simulink model "c00017M_harness"  (R2018a)
settings: Solver=FixedStepAuto  StartTime=0.0  StopTime=300  FixedStep=0.1  RelTol=1e-3
undefined symbols (not defined in the file): A1, hmax, R1, R2, sigbuilder_block
(part 2 of 6)

== system c00017M_harness/M127 ==
  note: VALUES
      | ---------------------------------
      | ControlType = 1 | 2 | 3
      | FillTank = 0 | 1
      | EmptyTank = 0 | 1
      | ManualReference between 0 and 1
      | Tempreature between 0 and 100
      | EmergencyButton = 0 | 1
      | LiquidLevel between 0 and 1 (hmax)
  note: Inputs For Tank2
  note: NAMES
      | --------------------------------------------
      | CT1 = ControlType Tank 1
      | F1 = Fill Tank 1
      | E1 = Empty Tank 1
      | MR1 = Manual Reference Tank1
      | T1 = Temperature Tank 1
      | EB1 = Emergency Button Tank 1
      | LL1 = Liquid Level 1
  note: Inputs For Tank3
  note: Inputs For Tank1
  CT2 : Inport
  F2 : Inport  Port=2
  E2 : Inport  Port=3
  MR2 : Inport  Port=4
  T2 : Inport  Port=5
  EB2 : Inport  Port=6
  Tank2 : Subsystem
  LL2 : Outport
  wires:
  Tank2/1(LL2) -> LL2/1
  EB2/1 -> Tank2/6(EB2)
  CT2/1 -> Tank2/1(CT2)
  F2/1 -> Tank2/2(F2)
  E2/1 -> Tank2/3(E2)
  T2/1 -> Tank2/5(T2)
  MR2/1 -> Tank2/4(MR2)

== system c00017M_harness/M128 ==
  note: VALUES
      | ---------------------------------
      | ControlType = 1 | 2 | 3
      | FillTank = 0 | 1
      | EmptyTank = 0 | 1
      | ManualReference between 0 and 1
      | Tempreature between 0 and 100
      | EmergencyButton = 0 | 1
      | LiquidLevel between 0 and 1 (hmax)
  note: Inputs For Tank2
  note: NAMES
      | --------------------------------------------
      | CT1 = ControlType Tank 1
      | F1 = Fill Tank 1
      | E1 = Empty Tank 1
      | MR1 = Manual Reference Tank1
      | T1 = Temperature Tank 1
      | EB1 = Emergency Button Tank 1
      | LL1 = Liquid Level 1
  note: Inputs For Tank3
  note: Inputs For Tank1
  CT2 : Inport
  F2 : Inport  Port=2
  E2 : Inport  Port=3
  MR2 : Inport  Port=4
  T2 : Inport  Port=5
  EB2 : Inport  Port=6
  Tank2 : Subsystem
  LL2 : Outport
  wires:
  Tank2/1(LL2) -> LL2/1
  EB2/1 -> Tank2/6(EB2)
  CT2/1 -> Tank2/1(CT2)
  F2/1 -> Tank2/2(F2)
  E2/1 -> Tank2/3(E2)
  T2/1 -> Tank2/5(T2)
  MR2/1 -> Tank2/4(MR2)

== system c00017M_harness/M129 ==
  note: VALUES
      | ---------------------------------
      | ControlType = 1 | 2 | 3
      | FillTank = 0 | 1
      | EmptyTank = 0 | 1
      | ManualReference between 0 and 1
      | Tempreature between 0 and 100
      | EmergencyButton = 0 | 1
      | LiquidLevel between 0 and 1 (hmax)
  note: Inputs For Tank2
  note: NAMES
      | --------------------------------------------
      | CT1 = ControlType Tank 1
      | F1 = Fill Tank 1
      | E1 = Empty Tank 1
      | MR1 = Manual Reference Tank1
      | T1 = Temperature Tank 1
      | EB1 = Emergency Button Tank 1
      | LL1 = Liquid Level 1
  note: Inputs For Tank3
  note: Inputs For Tank1
  CT2 : Inport
  F2 : Inport  Port=2
  E2 : Inport  Port=3
  MR2 : Inport  Port=4
  T2 : Inport  Port=5
  EB2 : Inport  Port=6
  Tank2 : Subsystem
  LL2 : Outport
  wires:
  Tank2/1(LL2) -> LL2/1
  EB2/1 -> Tank2/6(EB2)
  CT2/1 -> Tank2/1(CT2)
  F2/1 -> Tank2/2(F2)
  E2/1 -> Tank2/3(E2)
  T2/1 -> Tank2/5(T2)
  MR2/1 -> Tank2/4(MR2)

== system c00017M_harness/M130 ==
  note: VALUES
      | ---------------------------------
      | ControlType = 1 | 2 | 3
      | FillTank = 0 | 1
      | EmptyTank = 0 | 1
      | ManualReference between 0 and 1
      | Tempreature between 0 and 100
      | EmergencyButton = 0 | 1
      | LiquidLevel between 0 and 1 (hmax)
  note: Inputs For Tank2
  note: NAMES
      | --------------------------------------------
      | CT1 = ControlType Tank 1
      | F1 = Fill Tank 1
      | E1 = Empty Tank 1
      | MR1 = Manual Reference Tank1
      | T1 = Temperature Tank 1
      | EB1 = Emergency Button Tank 1
      | LL1 = Liquid Level 1
  note: Inputs For Tank3
  note: Inputs For Tank1
  CT2 : Inport
  F2 : Inport  Port=2
  E2 : Inport  Port=3
  MR2 : Inport  Port=4
  T2 : Inport  Port=5
  EB2 : Inport  Port=6
  Tank2 : Subsystem
  LL2 : Outport
  wires:
  Tank2/1(LL2) -> LL2/1
  EB2/1 -> Tank2/6(EB2)
  CT2/1 -> Tank2/1(CT2)
  F2/1 -> Tank2/2(F2)
  E2/1 -> Tank2/3(E2)
  T2/1 -> Tank2/5(T2)
  MR2/1 -> Tank2/4(MR2)

== system c00017M_harness/M131 ==
  note: VALUES
      | ---------------------------------
      | ControlType = 1 | 2 | 3
      | FillTank = 0 | 1
      | EmptyTank = 0 | 1
      | ManualReference between 0 and 1
      | Tempreature between 0 and 100
      | EmergencyButton = 0 | 1
      | LiquidLevel between 0 and 1 (hmax)
  note: Inputs For Tank2
  note: NAMES
      | --------------------------------------------
      | CT1 = ControlType Tank 1
      | F1 = Fill Tank 1
      | E1 = Empty Tank 1
      | MR1 = Manual Reference Tank1
      | T1 = Temperature Tank 1
      | EB1 = Emergency Button Tank 1
      | LL1 = Liquid Level 1
  note: Inputs For Tank3
  note: Inputs For Tank1
  CT2 : Inport
  F2 : Inport  Port=2
  E2 : Inport  Port=3
  MR2 : Inport  Port=4
  T2 : Inport  Port=5
  EB2 : Inport  Port=6
  Tank2 : Subsystem
  LL2 : Outport
  wires:
  Tank2/1(LL2) -> LL2/1
  EB2/1 -> Tank2/6(EB2)
  CT2/1 -> Tank2/1(CT2)
  F2/1 -> Tank2/2(F2)
  E2/1 -> Tank2/3(E2)
  T2/1 -> Tank2/5(T2)
  MR2/1 -> Tank2/4(MR2)

== system c00017M_harness/M132 ==
  note: VALUES
      | ---------------------------------
      | ControlType = 1 | 2 | 3
      | FillTank = 0 | 1
      | EmptyTank = 0 | 1
      | ManualReference between 0 and 1
      | Tempreature between 0 and 100
      | EmergencyButton = 0 | 1
      | LiquidLevel between 0 and 1 (hmax)
  note: Inputs For Tank2
  note: NAMES
      | --------------------------------------------
      | CT1 = ControlType Tank 1
      | F1 = Fill Tank 1
      | E1 = Empty Tank 1
      | MR1 = Manual Reference Tank1
      | T1 = Temperature Tank 1
      | EB1 = Emergency Button Tank 1
      | LL1 = Liquid Level 1
  note: Inputs For Tank3
  note: Inputs For Tank1
  CT2 : Inport
  F2 : Inport  Port=2
  E2 : Inport  Port=3
  MR2 : Inport  Port=4
  T2 : Inport  Port=5
  EB2 : Inport  Port=6
  Tank2 : Subsystem
  LL2 : Outport
  wires:
  Tank2/1(LL2) -> LL2/1
  EB2/1 -> Tank2/6(EB2)
  CT2/1 -> Tank2/1(CT2)
  F2/1 -> Tank2/2(F2)
  E2/1 -> Tank2/3(E2)
  T2/1 -> Tank2/5(T2)
  MR2/1 -> Tank2/4(MR2)

== system c00017M_harness/M133 ==
  note: VALUES
      | ---------------------------------
      | ControlType = 1 | 2 | 3
      | FillTank = 0 | 1
      | EmptyTank = 0 | 1
      | ManualReference between 0 and 1
      | Tempreature between 0 and 100
      | EmergencyButton = 0 | 1
      | LiquidLevel between 0 and 1 (hmax)
  note: Inputs For Tank2
  note: NAMES
      | --------------------------------------------
      | CT1 = ControlType Tank 1
      | F1 = Fill Tank 1
      | E1 = Empty Tank 1
      | MR1 = Manual Reference Tank1
      | T1 = Temperature Tank 1
      | EB1 = Emergency Button Tank 1
      | LL1 = Liquid Level 1
  note: Inputs For Tank3
  note: Inputs For Tank1
  CT2 : Inport
  F2 : Inport  Port=2
  E2 : Inport  Port=3
  MR2 : Inport  Port=4
  T2 : Inport  Port=5
  EB2 : Inport  Port=6
  Tank2 : Subsystem
  LL2 : Outport
  wires:
  Tank2/1(LL2) -> LL2/1
  EB2/1 -> Tank2/6(EB2)
  CT2/1 -> Tank2/1(CT2)
  F2/1 -> Tank2/2(F2)
  E2/1 -> Tank2/3(E2)
  T2/1 -> Tank2/5(T2)
  MR2/1 -> Tank2/4(MR2)

== system c00017M_harness/M134 ==
  note: VALUES
      | ---------------------------------
      | ControlType = 1 | 2 | 3
      | FillTank = 0 | 1
      | EmptyTank = 0 | 1
      | ManualReference between 0 and 1
      | Tempreature between 0 and 100
      | EmergencyButton = 0 | 1
      | LiquidLevel between 0 and 1 (hmax)
  note: Inputs For Tank2
  note: NAMES
      | --------------------------------------------
      | CT1 = ControlType Tank 1
      | F1 = Fill Tank 1
      | E1 = Empty Tank 1
      | MR1 = Manual Reference Tank1
      | T1 = Temperature Tank 1
      | EB1 = Emergency Button Tank 1
      | LL1 = Liquid Level 1
  note: Inputs For Tank3
  note: Inputs For Tank1
  CT2 : Inport
  F2 : Inport  Port=2
  E2 : Inport  Port=3
  MR2 : Inport  Port=4
  T2 : Inport  Port=5
  EB2 : Inport  Port=6
  Tank2 : Subsystem
  LL2 : Outport
  wires:
  Tank2/1(LL2) -> LL2/1
  EB2/1 -> Tank2/6(EB2)
  CT2/1 -> Tank2/1(CT2)
  F2/1 -> Tank2/2(F2)
  E2/1 -> Tank2/3(E2)
  T2/1 -> Tank2/5(T2)
  MR2/1 -> Tank2/4(MR2)

== system c00017M_harness/M135 ==
  note: VALUES
      | ---------------------------------
      | ControlType = 1 | 2 | 3
      | FillTank = 0 | 1
      | EmptyTank = 0 | 1
      | ManualReference between 0 and 1
      | Tempreature between 0 and 100
      | EmergencyButton = 0 | 1
      | LiquidLevel between 0 and 1 (hmax)
  note: Inputs For Tank2
  note: NAMES
      | --------------------------------------------
      | CT1 = ControlType Tank 1
      | F1 = Fill Tank 1
      | E1 = Empty Tank 1
      | MR1 = Manual Reference Tank1
      | T1 = Temperature Tank 1
      | EB1 = Emergency Button Tank 1
      | LL1 = Liquid Level 1
  note: Inputs For Tank3
  note: Inputs For Tank1
  CT2 : Inport
  F2 : Inport  Port=2
  E2 : Inport  Port=3
  MR2 : Inport  Port=4
  T2 : Inport  Port=5
  EB2 : Inport  Port=6
  Tank2 : Subsystem
  LL2 : Outport
  wires:
  Tank2/1(LL2) -> LL2/1
  EB2/1 -> Tank2/6(EB2)
  CT2/1 -> Tank2/1(CT2)
  F2/1 -> Tank2/2(F2)
  E2/1 -> Tank2/3(E2)
  T2/1 -> Tank2/5(T2)
  MR2/1 -> Tank2/4(MR2)

== system c00017M_harness/M136 ==
  note: VALUES
      | ---------------------------------
      | ControlType = 1 | 2 | 3
      | FillTank = 0 | 1
      | EmptyTank = 0 | 1
      | ManualReference between 0 and 1
      | Tempreature between 0 and 100
      | EmergencyButton = 0 | 1
      | LiquidLevel between 0 and 1 (hmax)
  note: Inputs For Tank2
  note: NAMES
      | --------------------------------------------
      | CT1 = ControlType Tank 1
      | F1 = Fill Tank 1
      | E1 = Empty Tank 1
      | MR1 = Manual Reference Tank1
      | T1 = Temperature Tank 1
      | EB1 = Emergency Button Tank 1
      | LL1 = Liquid Level 1
  note: Inputs For Tank3
  note: Inputs For Tank1
  CT2 : Inport
  F2 : Inport  Port=2
  E2 : Inport  Port=3
  MR2 : Inport  Port=4
  T2 : Inport  Port=5
  EB2 : Inport  Port=6
  Tank2 : Subsystem
  LL2 : Outport
  wires:
  Tank2/1(LL2) -> LL2/1
  EB2/1 -> Tank2/6(EB2)
  CT2/1 -> Tank2/1(CT2)
  F2/1 -> Tank2/2(F2)
  E2/1 -> Tank2/3(E2)
  T2/1 -> Tank2/5(T2)
  MR2/1 -> Tank2/4(MR2)

== system c00017M_harness/M137 ==
  note: VALUES
      | ---------------------------------
      | ControlType = 1 | 2 | 3
      | FillTank = 0 | 1
      | EmptyTank = 0 | 1
      | ManualReference between 0 and 1
      | Tempreature between 0 and 100
      | EmergencyButton = 0 | 1
      | LiquidLevel between 0 and 1 (hmax)
  note: Inputs For Tank2
  note: NAMES
      | --------------------------------------------
      | CT1 = ControlType Tank 1
      | F1 = Fill Tank 1
      | E1 = Empty Tank 1
      | MR1 = Manual Reference Tank1
      | T1 = Temperature Tank 1
      | EB1 = Emergency Button Tank 1
      | LL1 = Liquid Level 1
  note: Inputs For Tank3
  note: Inputs For Tank1
  CT2 : Inport
  F2 : Inport  Port=2
  E2 : Inport  Port=3
  MR2 : Inport  Port=4
  T2 : Inport  Port=5
  EB2 : Inport  Port=6
  Tank2 : Subsystem
  LL2 : Outport
  wires:
  Tank2/1(LL2) -> LL2/1
  EB2/1 -> Tank2/6(EB2)
  CT2/1 -> Tank2/1(CT2)
  F2/1 -> Tank2/2(F2)
  E2/1 -> Tank2/3(E2)
  T2/1 -> Tank2/5(T2)
  MR2/1 -> Tank2/4(MR2)

== system c00017M_harness/M138 ==
  note: VALUES
      | ---------------------------------
      | ControlType = 1 | 2 | 3
      | FillTank = 0 | 1
      | EmptyTank = 0 | 1
      | ManualReference between 0 and 1
      | Tempreature between 0 and 100
      | EmergencyButton = 0 | 1
      | LiquidLevel between 0 and 1 (hmax)
  note: Inputs For Tank2
  note: NAMES
      | --------------------------------------------
      | CT1 = ControlType Tank 1
      | F1 = Fill Tank 1
      | E1 = Empty Tank 1
      | MR1 = Manual Reference Tank1
      | T1 = Temperature Tank 1
      | EB1 = Emergency Button Tank 1
      | LL1 = Liquid Level 1
  note: Inputs For Tank3
  note: Inputs For Tank1
  CT2 : Inport
  F2 : Inport  Port=2
  E2 : Inport  Port=3
  MR2 : Inport  Port=4
  T2 : Inport  Port=5
  EB2 : Inport  Port=6
  Tank2 : Subsystem
  LL2 : Outport
  wires:
  Tank2/1(LL2) -> LL2/1
  EB2/1 -> Tank2/6(EB2)
  CT2/1 -> Tank2/1(CT2)
  F2/1 -> Tank2/2(F2)
  E2/1 -> Tank2/3(E2)
  T2/1 -> Tank2/5(T2)
  MR2/1 -> Tank2/4(MR2)

== system c00017M_harness/M140 ==
  note: VALUES
      | ---------------------------------
      | ControlType = 1 | 2 | 3
      | FillTank = 0 | 1
      | EmptyTank = 0 | 1
      | ManualReference between 0 and 1
      | Tempreature between 0 and 100
      | EmergencyButton = 0 | 1
      | LiquidLevel between 0 and 1 (hmax)
  note: Inputs For Tank2
  note: NAMES
      | --------------------------------------------
      | CT1 = ControlType Tank 1
      | F1 = Fill Tank 1
      | E1 = Empty Tank 1
      | MR1 = Manual Reference Tank1
      | T1 = Temperature Tank 1
      | EB1 = Emergency Button Tank 1
      | LL1 = Liquid Level 1
  note: Inputs For Tank3
  note: Inputs For Tank1
  CT2 : Inport
  F2 : Inport  Port=2
  E2 : Inport  Port=3
  MR2 : Inport  Port=4
  T2 : Inport  Port=5
  EB2 : Inport  Port=6
  Tank2 : Subsystem
  LL2 : Outport
  wires:
  Tank2/1(LL2) -> LL2/1
  EB2/1 -> Tank2/6(EB2)
  CT2/1 -> Tank2/1(CT2)
  F2/1 -> Tank2/2(F2)
  E2/1 -> Tank2/3(E2)
  T2/1 -> Tank2/5(T2)
  MR2/1 -> Tank2/4(MR2)

== system c00017M_harness/M141 ==
  note: VALUES
      | ---------------------------------
      | ControlType = 1 | 2 | 3
      | FillTank = 0 | 1
      | EmptyTank = 0 | 1
      | ManualReference between 0 and 1
      | Tempreature between 0 and 100
      | EmergencyButton = 0 | 1
      | LiquidLevel between 0 and 1 (hmax)
  note: Inputs For Tank2
  note: NAMES
      | --------------------------------------------
      | CT1 = ControlType Tank 1
      | F1 = Fill Tank 1
      | E1 = Empty Tank 1
      | MR1 = Manual Reference Tank1
      | T1 = Temperature Tank 1
      | EB1 = Emergency Button Tank 1
      | LL1 = Liquid Level 1
  note: Inputs For Tank3
  note: Inputs For Tank1
  CT2 : Inport
  F2 : Inport  Port=2
  E2 : Inport  Port=3
  MR2 : Inport  Port=4
  T2 : Inport  Port=5
  EB2 : Inport  Port=6
  Tank2 : Subsystem
  LL2 : Outport
  wires:
  Tank2/1(LL2) -> LL2/1
  EB2/1 -> Tank2/6(EB2)
  CT2/1 -> Tank2/1(CT2)
  F2/1 -> Tank2/2(F2)
  E2/1 -> Tank2/3(E2)
  T2/1 -> Tank2/5(T2)
  MR2/1 -> Tank2/4(MR2)

== system c00017M_harness/M142 ==
  note: VALUES
      | ---------------------------------
      | ControlType = 1 | 2 | 3
      | FillTank = 0 | 1
      | EmptyTank = 0 | 1
      | ManualReference between 0 and 1
      | Tempreature between 0 and 100
      | EmergencyButton = 0 | 1
      | LiquidLevel between 0 and 1 (hmax)
  note: Inputs For Tank2
  note: NAMES
      | --------------------------------------------
      | CT1 = ControlType Tank 1
      | F1 = Fill Tank 1
      | E1 = Empty Tank 1
      | MR1 = Manual Reference Tank1
      | T1 = Temperature Tank 1
      | EB1 = Emergency Button Tank 1
      | LL1 = Liquid Level 1
  note: Inputs For Tank3
  note: Inputs For Tank1
  CT2 : Inport
  F2 : Inport  Port=2
  E2 : Inport  Port=3
  MR2 : Inport  Port=4
  T2 : Inport  Port=5
  EB2 : Inport  Port=6
  Tank2 : Subsystem
  LL2 : Outport
  wires:
  Tank2/1(LL2) -> LL2/1
  EB2/1 -> Tank2/6(EB2)
  CT2/1 -> Tank2/1(CT2)
  F2/1 -> Tank2/2(F2)
  E2/1 -> Tank2/3(E2)
  T2/1 -> Tank2/5(T2)
  MR2/1 -> Tank2/4(MR2)

== system c00017M_harness/M143 ==
  note: VALUES
      | ---------------------------------
      | ControlType = 1 | 2 | 3
      | FillTank = 0 | 1
      | EmptyTank = 0 | 1
      | ManualReference between 0 and 1
      | Tempreature between 0 and 100
      | EmergencyButton = 0 | 1
      | LiquidLevel between 0 and 1 (hmax)
  note: Inputs For Tank2
  note: NAMES
      | --------------------------------------------
      | CT1 = ControlType Tank 1
      | F1 = Fill Tank 1
      | E1 = Empty Tank 1
      | MR1 = Manual Reference Tank1
      | T1 = Temperature Tank 1
      | EB1 = Emergency Button Tank 1
      | LL1 = Liquid Level 1
  note: Inputs For Tank3
  note: Inputs For Tank1
  CT2 : Inport
  F2 : Inport  Port=2
  E2 : Inport  Port=3
  MR2 : Inport  Port=4
  T2 : Inport  Port=5
  EB2 : Inport  Port=6
  Tank2 : Subsystem
  LL2 : Outport
  wires:
  Tank2/1(LL2) -> LL2/1
  EB2/1 -> Tank2/6(EB2)
  CT2/1 -> Tank2/1(CT2)
  F2/1 -> Tank2/2(F2)
  E2/1 -> Tank2/3(E2)
  T2/1 -> Tank2/5(T2)
  MR2/1 -> Tank2/4(MR2)

== system c00017M_harness/M151 ==
  note: VALUES
      | ---------------------------------
      | ControlType = 1 | 2 | 3
      | FillTank = 0 | 1
      | EmptyTank = 0 | 1
      | ManualReference between 0 and 1
      | Tempreature between 0 and 100
      | EmergencyButton = 0 | 1
      | LiquidLevel between 0 and 1 (hmax)
  note: Inputs For Tank2
  note: NAMES
      | --------------------------------------------
      | CT1 = ControlType Tank 1
      | F1 = Fill Tank 1
      | E1 = Empty Tank 1
      | MR1 = Manual Reference Tank1
      | T1 = Temperature Tank 1
      | EB1 = Emergency Button Tank 1
      | LL1 = Liquid Level 1
  note: Inputs For Tank3
  note: Inputs For Tank1
  CT2 : Inport
  F2 : Inport  Port=2
  E2 : Inport  Port=3
  MR2 : Inport  Port=4
  T2 : Inport  Port=5
  EB2 : Inport  Port=6
  Tank2 : Subsystem
  LL2 : Outport
  wires:
  Tank2/1(LL2) -> LL2/1
  EB2/1 -> Tank2/6(EB2)
  CT2/1 -> Tank2/1(CT2)
  F2/1 -> Tank2/2(F2)
  E2/1 -> Tank2/3(E2)
  T2/1 -> Tank2/5(T2)
  MR2/1 -> Tank2/4(MR2)

== system c00017M_harness/M152 ==
  note: VALUES
      | ---------------------------------
      | ControlType = 1 | 2 | 3
      | FillTank = 0 | 1
      | EmptyTank = 0 | 1
      | ManualReference between 0 and 1
      | Tempreature between 0 and 100
      | EmergencyButton = 0 | 1
      | LiquidLevel between 0 and 1 (hmax)
  note: Inputs For Tank2
  note: NAMES
      | --------------------------------------------
      | CT1 = ControlType Tank 1
      | F1 = Fill Tank 1
      | E1 = Empty Tank 1
      | MR1 = Manual Reference Tank1
      | T1 = Temperature Tank 1
      | EB1 = Emergency Button Tank 1
      | LL1 = Liquid Level 1
  note: Inputs For Tank3
  note: Inputs For Tank1
  CT2 : Inport
  F2 : Inport  Port=2
  E2 : Inport  Port=3
  MR2 : Inport  Port=4
  T2 : Inport  Port=5
  EB2 : Inport  Port=6
  Tank2 : Subsystem
  LL2 : Outport
  wires:
  Tank2/1(LL2) -> LL2/1
  EB2/1 -> Tank2/6(EB2)
  CT2/1 -> Tank2/1(CT2)
  F2/1 -> Tank2/2(F2)
  E2/1 -> Tank2/3(E2)
  T2/1 -> Tank2/5(T2)
  MR2/1 -> Tank2/4(MR2)

== system c00017M_harness/M153 ==
  note: VALUES
      | ---------------------------------
      | ControlType = 1 | 2 | 3
      | FillTank = 0 | 1
      | EmptyTank = 0 | 1
      | ManualReference between 0 and 1
      | Tempreature between 0 and 100
      | EmergencyButton = 0 | 1
      | LiquidLevel between 0 and 1 (hmax)
  note: Inputs For Tank2
  note: NAMES
      | --------------------------------------------
      | CT1 = ControlType Tank 1
      | F1 = Fill Tank 1
      | E1 = Empty Tank 1
      | MR1 = Manual Reference Tank1
      | T1 = Temperature Tank 1
      | EB1 = Emergency Button Tank 1
      | LL1 = Liquid Level 1
  note: Inputs For Tank3
  note: Inputs For Tank1
  CT2 : Inport
  F2 : Inport  Port=2
  E2 : Inport  Port=3
  MR2 : Inport  Port=4
  T2 : Inport  Port=5
  EB2 : Inport  Port=6
  Tank2 : Subsystem
  LL2 : Outport
  wires:
  Tank2/1(LL2) -> LL2/1
  EB2/1 -> Tank2/6(EB2)
  CT2/1 -> Tank2/1(CT2)
  F2/1 -> Tank2/2(F2)
  E2/1 -> Tank2/3(E2)
  T2/1 -> Tank2/5(T2)
  MR2/1 -> Tank2/4(MR2)

== system c00017M_harness/M154 ==
  note: VALUES
      | ---------------------------------
      | ControlType = 1 | 2 | 3
      | FillTank = 0 | 1
      | EmptyTank = 0 | 1
      | ManualReference between 0 and 1
      | Tempreature between 0 and 100
      | EmergencyButton = 0 | 1
      | LiquidLevel between 0 and 1 (hmax)
  note: Inputs For Tank2
  note: NAMES
      | --------------------------------------------
      | CT1 = ControlType Tank 1
      | F1 = Fill Tank 1
      | E1 = Empty Tank 1
      | MR1 = Manual Reference Tank1
      | T1 = Temperature Tank 1
      | EB1 = Emergency Button Tank 1
      | LL1 = Liquid Level 1
  note: Inputs For Tank3
  note: Inputs For Tank1
  CT2 : Inport
  F2 : Inport  Port=2
  E2 : Inport  Port=3
  MR2 : Inport  Port=4
  T2 : Inport  Port=5
  EB2 : Inport  Port=6
  Tank2 : Subsystem
  LL2 : Outport
  wires:
  Tank2/1(LL2) -> LL2/1
  EB2/1 -> Tank2/6(EB2)
  CT2/1 -> Tank2/1(CT2)
  F2/1 -> Tank2/2(F2)
  E2/1 -> Tank2/3(E2)
  T2/1 -> Tank2/5(T2)
  MR2/1 -> Tank2/4(MR2)

== system c00017M_harness/M155 ==
  note: VALUES
      | ---------------------------------
      | ControlType = 1 | 2 | 3
      | FillTank = 0 | 1
      | EmptyTank = 0 | 1
      | ManualReference between 0 and 1
      | Tempreature between 0 and 100
      | EmergencyButton = 0 | 1
      | LiquidLevel between 0 and 1 (hmax)
  note: Inputs For Tank2
  note: NAMES
      | --------------------------------------------
      | CT1 = ControlType Tank 1
      | F1 = Fill Tank 1
      | E1 = Empty Tank 1
      | MR1 = Manual Reference Tank1
      | T1 = Temperature Tank 1
      | EB1 = Emergency Button Tank 1
      | LL1 = Liquid Level 1
  note: Inputs For Tank3
  note: Inputs For Tank1
  CT2 : Inport
  F2 : Inport  Port=2
  E2 : Inport  Port=3
  MR2 : Inport  Port=4
  T2 : Inport  Port=5
  EB2 : Inport  Port=6
  Tank2 : Subsystem
  LL2 : Outport
  wires:
  Tank2/1(LL2) -> LL2/1
  EB2/1 -> Tank2/6(EB2)
  CT2/1 -> Tank2/1(CT2)
  F2/1 -> Tank2/2(F2)
  E2/1 -> Tank2/3(E2)
  T2/1 -> Tank2/5(T2)
  MR2/1 -> Tank2/4(MR2)

== system c00017M_harness/M156 ==
  note: VALUES
      | ---------------------------------
      | ControlType = 1 | 2 | 3
      | FillTank = 0 | 1
      | EmptyTank = 0 | 1
      | ManualReference between 0 and 1
      | Tempreature between 0 and 100
      | EmergencyButton = 0 | 1
      | LiquidLevel between 0 and 1 (hmax)
  note: Inputs For Tank2
  note: NAMES
      | --------------------------------------------
      | CT1 = ControlType Tank 1
      | F1 = Fill Tank 1
      | E1 = Empty Tank 1
      | MR1 = Manual Reference Tank1
      | T1 = Temperature Tank 1
      | EB1 = Emergency Button Tank 1
      | LL1 = Liquid Level 1
  note: Inputs For Tank3
  note: Inputs For Tank1
  CT2 : Inport
  F2 : Inport  Port=2
  E2 : Inport  Port=3
  MR2 : Inport  Port=4
  T2 : Inport  Port=5
  EB2 : Inport  Port=6
  Tank2 : Subsystem
  LL2 : Outport
  wires:
  Tank2/1(LL2) -> LL2/1
  EB2/1 -> Tank2/6(EB2)
  CT2/1 -> Tank2/1(CT2)
  F2/1 -> Tank2/2(F2)
  E2/1 -> Tank2/3(E2)
  T2/1 -> Tank2/5(T2)
  MR2/1 -> Tank2/4(MR2)

== system c00017M_harness/M157 ==
  note: VALUES
      | ---------------------------------
      | ControlType = 1 | 2 | 3
      | FillTank = 0 | 1
      | EmptyTank = 0 | 1
      | ManualReference between 0 and 1
      | Tempreature between 0 and 100
      | EmergencyButton = 0 | 1
      | LiquidLevel between 0 and 1 (hmax)
  note: Inputs For Tank2
  note: NAMES
      | --------------------------------------------
      | CT1 = ControlType Tank 1
      | F1 = Fill Tank 1
      | E1 = Empty Tank 1
      | MR1 = Manual Reference Tank1
      | T1 = Temperature Tank 1
      | EB1 = Emergency Button Tank 1
      | LL1 = Liquid Level 1
  note: Inputs For Tank3
  note: Inputs For Tank1
  CT2 : Inport
  F2 : Inport  Port=2
  E2 : Inport  Port=3
  MR2 : Inport  Port=4
  T2 : Inport  Port=5
  EB2 : Inport  Port=6
  Tank2 : Subsystem
  LL2 : Outport
  wires:
  Tank2/1(LL2) -> LL2/1
  EB2/1 -> Tank2/6(EB2)
  CT2/1 -> Tank2/1(CT2)
  F2/1 -> Tank2/2(F2)
  E2/1 -> Tank2/3(E2)
  T2/1 -> Tank2/5(T2)
  MR2/1 -> Tank2/4(MR2)

== system c00017M_harness/M158 ==
  note: VALUES
      | ---------------------------------
      | ControlType = 1 | 2 | 3
      | FillTank = 0 | 1
      | EmptyTank = 0 | 1
      | ManualReference between 0 and 1
      | Tempreature between 0 and 100
      | EmergencyButton = 0 | 1
      | LiquidLevel between 0 and 1 (hmax)
  note: Inputs For Tank2
  note: NAMES
      | --------------------------------------------
      | CT1 = ControlType Tank 1
      | F1 = Fill Tank 1
      | E1 = Empty Tank 1
      | MR1 = Manual Reference Tank1
      | T1 = Temperature Tank 1
      | EB1 = Emergency Button Tank 1
      | LL1 = Liquid Level 1
  note: Inputs For Tank3
  note: Inputs For Tank1
  CT2 : Inport
  F2 : Inport  Port=2
  E2 : Inport  Port=3
  MR2 : Inport  Port=4
  T2 : Inport  Port=5
  EB2 : Inport  Port=6
  Tank2 : Subsystem
  LL2 : Outport
  wires:
  Tank2/1(LL2) -> LL2/1
  EB2/1 -> Tank2/6(EB2)
  CT2/1 -> Tank2/1(CT2)
  F2/1 -> Tank2/2(F2)
  E2/1 -> Tank2/3(E2)
  T2/1 -> Tank2/5(T2)
  MR2/1 -> Tank2/4(MR2)

== system c00017M_harness/M159 ==
  note: VALUES
      | ---------------------------------
      | ControlType = 1 | 2 | 3
      | FillTank = 0 | 1
      | EmptyTank = 0 | 1
      | ManualReference between 0 and 1
      | Tempreature between 0 and 100
      | EmergencyButton = 0 | 1
      | LiquidLevel between 0 and 1 (hmax)
  note: Inputs For Tank2
  note: NAMES
      | --------------------------------------------
      | CT1 = ControlType Tank 1
      | F1 = Fill Tank 1
      | E1 = Empty Tank 1
      | MR1 = Manual Reference Tank1
      | T1 = Temperature Tank 1
      | EB1 = Emergency Button Tank 1
      | LL1 = Liquid Level 1
  note: Inputs For Tank3
  note: Inputs For Tank1
  CT2 : Inport
  F2 : Inport  Port=2
  E2 : Inport  Port=3
  MR2 : Inport  Port=4
  T2 : Inport  Port=5
  EB2 : Inport  Port=6
  Tank2 : Subsystem
  LL2 : Outport
  wires:
  Tank2/1(LL2) -> LL2/1
  EB2/1 -> Tank2/6(EB2)
  CT2/1 -> Tank2/1(CT2)
  F2/1 -> Tank2/2(F2)
  E2/1 -> Tank2/3(E2)
  T2/1 -> Tank2/5(T2)
  MR2/1 -> Tank2/4(MR2)

== system c00017M_harness/M160 ==
  note: VALUES
      | ---------------------------------
      | ControlType = 1 | 2 | 3
      | FillTank = 0 | 1
      | EmptyTank = 0 | 1
      | ManualReference between 0 and 1
      | Tempreature between 0 and 100
      | EmergencyButton = 0 | 1
      | LiquidLevel between 0 and 1 (hmax)
  note: Inputs For Tank2
  note: NAMES
      | --------------------------------------------
      | CT1 = ControlType Tank 1
      | F1 = Fill Tank 1
      | E1 = Empty Tank 1
      | MR1 = Manual Reference Tank1
      | T1 = Temperature Tank 1
      | EB1 = Emergency Button Tank 1
      | LL1 = Liquid Level 1
  note: Inputs For Tank3
  note: Inputs For Tank1
  CT2 : Inport
  F2 : Inport  Port=2
  E2 : Inport  Port=3
  MR2 : Inport  Port=4
  T2 : Inport  Port=5
  EB2 : Inport  Port=6
  Tank2 : Subsystem
  LL2 : Outport
  wires:
  Tank2/1(LL2) -> LL2/1
  EB2/1 -> Tank2/6(EB2)
  CT2/1 -> Tank2/1(CT2)
  F2/1 -> Tank2/2(F2)
  E2/1 -> Tank2/3(E2)
  T2/1 -> Tank2/5(T2)
  MR2/1 -> Tank2/4(MR2)

== system c00017M_harness/M161 ==
  note: VALUES
      | ---------------------------------
      | ControlType = 1 | 2 | 3
      | FillTank = 0 | 1
      | EmptyTank = 0 | 1
      | ManualReference between 0 and 1
      | Tempreature between 0 and 100
      | EmergencyButton = 0 | 1
      | LiquidLevel between 0 and 1 (hmax)
  note: Inputs For Tank2
  note: NAMES
      | --------------------------------------------
      | CT1 = ControlType Tank 1
      | F1 = Fill Tank 1
      | E1 = Empty Tank 1
      | MR1 = Manual Reference Tank1
      | T1 = Temperature Tank 1
      | EB1 = Emergency Button Tank 1
      | LL1 = Liquid Level 1
  note: Inputs For Tank3
  note: Inputs For Tank1
  CT2 : Inport
  F2 : Inport  Port=2
  E2 : Inport  Port=3
  MR2 : Inport  Port=4
  T2 : Inport  Port=5
  EB2 : Inport  Port=6
  Tank2 : Subsystem
  LL2 : Outport
  wires:
  Tank2/1(LL2) -> LL2/1
  EB2/1 -> Tank2/6(EB2)
  CT2/1 -> Tank2/1(CT2)
  F2/1 -> Tank2/2(F2)
  E2/1 -> Tank2/3(E2)
  T2/1 -> Tank2/5(T2)
  MR2/1 -> Tank2/4(MR2)

== system c00017M_harness/M162 ==
  note: VALUES
      | ---------------------------------
      | ControlType = 1 | 2 | 3
      | FillTank = 0 | 1
      | EmptyTank = 0 | 1
      | ManualReference between 0 and 1
      | Tempreature between 0 and 100
      | EmergencyButton = 0 | 1
      | LiquidLevel between 0 and 1 (hmax)
  note: Inputs For Tank2
  note: NAMES
      | --------------------------------------------
      | CT1 = ControlType Tank 1
      | F1 = Fill Tank 1
      | E1 = Empty Tank 1
      | MR1 = Manual Reference Tank1
      | T1 = Temperature Tank 1
      | EB1 = Emergency Button Tank 1
      | LL1 = Liquid Level 1
  note: Inputs For Tank3
  note: Inputs For Tank1
  CT2 : Inport
  F2 : Inport  Port=2
  E2 : Inport  Port=3
  MR2 : Inport  Port=4
  T2 : Inport  Port=5
  EB2 : Inport  Port=6
  Tank2 : Subsystem
  LL2 : Outport
  wires:
  Tank2/1(LL2) -> LL2/1
  EB2/1 -> Tank2/6(EB2)
  CT2/1 -> Tank2/1(CT2)
  F2/1 -> Tank2/2(F2)
  E2/1 -> Tank2/3(E2)
  T2/1 -> Tank2/5(T2)
  MR2/1 -> Tank2/4(MR2)

== system c00017M_harness/M163 ==
  note: VALUES
      | ---------------------------------
      | ControlType = 1 | 2 | 3
      | FillTank = 0 | 1
      | EmptyTank = 0 | 1
      | ManualReference between 0 and 1
      | Tempreature between 0 and 100
      | EmergencyButton = 0 | 1
      | LiquidLevel between 0 and 1 (hmax)
  note: Inputs For Tank2
  note: NAMES
      | --------------------------------------------
      | CT1 = ControlType Tank 1
      | F1 = Fill Tank 1
      | E1 = Empty Tank 1
      | MR1 = Manual Reference Tank1
      | T1 = Temperature Tank 1
      | EB1 = Emergency Button Tank 1
      | LL1 = Liquid Level 1
  note: Inputs For Tank3
  note: Inputs For Tank1
  CT2 : Inport
  F2 : Inport  Port=2
  E2 : Inport  Port=3
  MR2 : Inport  Port=4
  T2 : Inport  Port=5
  EB2 : Inport  Port=6
  Tank2 : Subsystem
  LL2 : Outport
  wires:
  Tank2/1(LL2) -> LL2/1
  EB2/1 -> Tank2/6(EB2)
  CT2/1 -> Tank2/1(CT2)
  F2/1 -> Tank2/2(F2)
  E2/1 -> Tank2/3(E2)
  T2/1 -> Tank2/5(T2)
  MR2/1 -> Tank2/4(MR2)

== system c00017M_harness/M164 ==
  note: VALUES
      | ---------------------------------
      | ControlType = 1 | 2 | 3
      | FillTank = 0 | 1
      | EmptyTank = 0 | 1
      | ManualReference between 0 and 1
      | Tempreature between 0 and 100
      | EmergencyButton = 0 | 1
      | LiquidLevel between 0 and 1 (hmax)
  note: Inputs For Tank2
  note: NAMES
      | --------------------------------------------
      | CT1 = ControlType Tank 1
      | F1 = Fill Tank 1
      | E1 = Empty Tank 1
      | MR1 = Manual Reference Tank1
      | T1 = Temperature Tank 1
      | EB1 = Emergency Button Tank 1
      | LL1 = Liquid Level 1
  note: Inputs For Tank3
  note: Inputs For Tank1
  CT2 : Inport
  F2 : Inport  Port=2
  E2 : Inport  Port=3
  MR2 : Inport  Port=4
  T2 : Inport  Port=5
  EB2 : Inport  Port=6
  Tank2 : Subsystem
  LL2 : Outport
  wires:
  Tank2/1(LL2) -> LL2/1
  EB2/1 -> Tank2/6(EB2)
  CT2/1 -> Tank2/1(CT2)
  F2/1 -> Tank2/2(F2)
  E2/1 -> Tank2/3(E2)
  T2/1 -> Tank2/5(T2)
  MR2/1 -> Tank2/4(MR2)

== system c00017M_harness/CPSUT/Tank2 ==
  CT2 : Inport
  F2 : Inport  Port=2
  E2 : Inport  Port=3
  MR2 : Inport  Port=4
  T2 : Inport  Port=5
  EB2 : Inport  Port=6
  Control : Subsystem
  Memory : Memory
  TankModel : Subsystem
  LL2 : Outport
  wires:
  TankModel/1(LiquidLevel) -> Memory/1, LL2/1
  Control/2(LiquidOut) -> TankModel/2(LiquidOut)
  Memory/1 -> Control/6(LiquidLevel)
  MR2/1 -> Control/2(ManualReference)
  CT2/1 -> Control/1(ControlType)
  F2/1 -> Control/3(Fill)
  E2/1 -> Control/4(Empty)
  EB2/1 -> Control/5(EmergencyButton)
  Control/1(LiquidIn) -> TankModel/1(LiquidIn)

== system c00017M_harness/M083/Tank2 ==
  CT2 : Inport
  F2 : Inport  Port=2
  E2 : Inport  Port=3
  MR2 : Inport  Port=4
  T2 : Inport  Port=5
  EB2 : Inport  Port=6
  Control : Subsystem
  Memory : Memory
  TankModel : Subsystem
  LL2 : Outport
  wires:
  TankModel/1(LiquidLevel) -> Memory/1, LL2/1
  Control/2(LiquidOut) -> TankModel/2(LiquidOut)
  Memory/1 -> Control/6(LiquidLevel)
  MR2/1 -> Control/2(ManualReference)
  CT2/1 -> Control/1(ControlType)
  F2/1 -> Control/3(Fill)
  E2/1 -> Control/4(Empty)
  EB2/1 -> Control/5(EmergencyButton)
  Control/1(LiquidIn) -> TankModel/1(LiquidIn)

== system c00017M_harness/M118/Tank2 ==
  CT2 : Inport
  F2 : Inport  Port=2
  E2 : Inport  Port=3
  MR2 : Inport  Port=4
  T2 : Inport  Port=5
  EB2 : Inport  Port=6
  Control : Subsystem
  Memory : Memory
  TankModel : Subsystem
  LL2 : Outport
  wires:
  TankModel/1(LiquidLevel) -> Memory/1, LL2/1
  Control/2(LiquidOut) -> TankModel/2(LiquidOut)
  Memory/1 -> Control/6(LiquidLevel)
  MR2/1 -> Control/2(ManualReference)
  CT2/1 -> Control/1(ControlType)
  F2/1 -> Control/3(Fill)
  E2/1 -> Control/4(Empty)
  EB2/1 -> Control/5(EmergencyButton)
  Control/1(LiquidIn) -> TankModel/1(LiquidIn)

== system c00017M_harness/M119/Tank2 ==
  CT2 : Inport
  F2 : Inport  Port=2
  E2 : Inport  Port=3
  MR2 : Inport  Port=4
  T2 : Inport  Port=5
  EB2 : Inport  Port=6
  Control : Subsystem
  Memory : Memory
  TankModel : Subsystem
  LL2 : Outport
  wires:
  TankModel/1(LiquidLevel) -> Memory/1, LL2/1
  Control/2(LiquidOut) -> TankModel/2(LiquidOut)
  Memory/1 -> Control/6(LiquidLevel)
  MR2/1 -> Control/2(ManualReference)
  CT2/1 -> Control/1(ControlType)
  F2/1 -> Control/3(Fill)
  E2/1 -> Control/4(Empty)
  EB2/1 -> Control/5(EmergencyButton)
  Control/1(LiquidIn) -> TankModel/1(LiquidIn)

== system c00017M_harness/M120/Tank2 ==
  CT2 : Inport
  F2 : Inport  Port=2
  E2 : Inport  Port=3
  MR2 : Inport  Port=4
  T2 : Inport  Port=5
  EB2 : Inport  Port=6
  Control : Subsystem
  Memory : Memory
  TankModel : Subsystem
  LL2 : Outport
  wires:
  TankModel/1(LiquidLevel) -> Memory/1, LL2/1
  Control/2(LiquidOut) -> TankModel/2(LiquidOut)
  Memory/1 -> Control/6(LiquidLevel)
  MR2/1 -> Control/2(ManualReference)
  CT2/1 -> Control/1(ControlType)
  F2/1 -> Control/3(Fill)
  E2/1 -> Control/4(Empty)
  EB2/1 -> Control/5(EmergencyButton)
  Control/1(LiquidIn) -> TankModel/1(LiquidIn)

== system c00017M_harness/M121/Tank2 ==
  CT2 : Inport
  F2 : Inport  Port=2
  E2 : Inport  Port=3
  MR2 : Inport  Port=4
  T2 : Inport  Port=5
  EB2 : Inport  Port=6
  Control : Subsystem
  Memory : Memory
  TankModel : Subsystem
  LL2 : Outport
  wires:
  TankModel/1(LiquidLevel) -> Memory/1, LL2/1
  Control/2(LiquidOut) -> TankModel/2(LiquidOut)
  Memory/1 -> Control/6(LiquidLevel)
  MR2/1 -> Control/2(ManualReference)
  CT2/1 -> Control/1(ControlType)
  F2/1 -> Control/3(Fill)
  E2/1 -> Control/4(Empty)
  EB2/1 -> Control/5(EmergencyButton)
  Control/1(LiquidIn) -> TankModel/1(LiquidIn)

== system c00017M_harness/M122/Tank2 ==
  CT2 : Inport
  F2 : Inport  Port=2
  E2 : Inport  Port=3
  MR2 : Inport  Port=4
  T2 : Inport  Port=5
  EB2 : Inport  Port=6
  Control : Subsystem
  Memory : Memory
  TankModel : Subsystem
  LL2 : Outport
  wires:
  TankModel/1(LiquidLevel) -> Memory/1, LL2/1
  Control/2(LiquidOut) -> TankModel/2(LiquidOut)
  Memory/1 -> Control/6(LiquidLevel)
  MR2/1 -> Control/2(ManualReference)
  CT2/1 -> Control/1(ControlType)
  F2/1 -> Control/3(Fill)
  E2/1 -> Control/4(Empty)
  EB2/1 -> Control/5(EmergencyButton)
  Control/1(LiquidIn) -> TankModel/1(LiquidIn)

== system c00017M_harness/M123/Tank2 ==
  CT2 : Inport
  F2 : Inport  Port=2
  E2 : Inport  Port=3
  MR2 : Inport  Port=4
  T2 : Inport  Port=5
  EB2 : Inport  Port=6
  Control : Subsystem
  Memory : Memory
  TankModel : Subsystem
  LL2 : Outport
  wires:
  TankModel/1(LiquidLevel) -> Memory/1, LL2/1
  Control/2(LiquidOut) -> TankModel/2(LiquidOut)
  Memory/1 -> Control/6(LiquidLevel)
  MR2/1 -> Control/2(ManualReference)
  CT2/1 -> Control/1(ControlType)
  F2/1 -> Control/3(Fill)
  E2/1 -> Control/4(Empty)
  EB2/1 -> Control/5(EmergencyButton)
  Control/1(LiquidIn) -> TankModel/1(LiquidIn)

== system c00017M_harness/M124/Tank2 ==
  CT2 : Inport
  F2 : Inport  Port=2
  E2 : Inport  Port=3
  MR2 : Inport  Port=4
  T2 : Inport  Port=5
  EB2 : Inport  Port=6
  Control : Subsystem
  Memory : Memory
  TankModel : Subsystem
  LL2 : Outport
  wires:
  TankModel/1(LiquidLevel) -> Memory/1, LL2/1
  Control/2(LiquidOut) -> TankModel/2(LiquidOut)
  Memory/1 -> Control/6(LiquidLevel)
  MR2/1 -> Control/2(ManualReference)
  CT2/1 -> Control/1(ControlType)
  F2/1 -> Control/3(Fill)
  E2/1 -> Control/4(Empty)
  EB2/1 -> Control/5(EmergencyButton)
  Control/1(LiquidIn) -> TankModel/1(LiquidIn)

== system c00017M_harness/M125/Tank2 ==
  CT2 : Inport
  F2 : Inport  Port=2
  E2 : Inport  Port=3
  MR2 : Inport  Port=4
  T2 : Inport  Port=5
  EB2 : Inport  Port=6
  Control : Subsystem
  Memory : Memory
  TankModel : Subsystem
  LL2 : Outport
  wires:
  TankModel/1(LiquidLevel) -> Memory/1, LL2/1
  Control/2(LiquidOut) -> TankModel/2(LiquidOut)
  Memory/1 -> Control/6(LiquidLevel)
  MR2/1 -> Control/2(ManualReference)
  CT2/1 -> Control/1(ControlType)
  F2/1 -> Control/3(Fill)
  E2/1 -> Control/4(Empty)
  EB2/1 -> Control/5(EmergencyButton)
  Control/1(LiquidIn) -> TankModel/1(LiquidIn)

== system c00017M_harness/M126/Tank2 ==
  CT2 : Inport
  F2 : Inport  Port=2
  E2 : Inport  Port=3
  MR2 : Inport  Port=4
  T2 : Inport  Port=5
  EB2 : Inport  Port=6
  Control : Subsystem
  Memory : Memory
  TankModel : Subsystem
  LL2 : Outport
  wires:
  TankModel/1(LiquidLevel) -> Memory/1, LL2/1
  Control/2(LiquidOut) -> TankModel/2(LiquidOut)
  Memory/1 -> Control/6(LiquidLevel)
  MR2/1 -> Control/2(ManualReference)
  CT2/1 -> Control/1(ControlType)
  F2/1 -> Control/3(Fill)
  E2/1 -> Control/4(Empty)
  EB2/1 -> Control/5(EmergencyButton)
  Control/1(LiquidIn) -> TankModel/1(LiquidIn)

== system c00017M_harness/M127/Tank2 ==
  CT2 : Inport
  F2 : Inport  Port=2
  E2 : Inport  Port=3
  MR2 : Inport  Port=4
  T2 : Inport  Port=5
  EB2 : Inport  Port=6
  Control : Subsystem
  Memory : Memory
  TankModel : Subsystem
  LL2 : Outport
  wires:
  TankModel/1(LiquidLevel) -> Memory/1, LL2/1
  Control/2(LiquidOut) -> TankModel/2(LiquidOut)
  Memory/1 -> Control/6(LiquidLevel)
  MR2/1 -> Control/2(ManualReference)
  CT2/1 -> Control/1(ControlType)
  F2/1 -> Control/3(Fill)
  E2/1 -> Control/4(Empty)
  EB2/1 -> Control/5(EmergencyButton)
  Control/1(LiquidIn) -> TankModel/1(LiquidIn)

== system c00017M_harness/M128/Tank2 ==
  CT2 : Inport
  F2 : Inport  Port=2
  E2 : Inport  Port=3
  MR2 : Inport  Port=4
  T2 : Inport  Port=5
  EB2 : Inport  Port=6
  Control : Subsystem
  Memory : Memory
  TankModel : Subsystem
  LL2 : Outport
  wires:
  TankModel/1(LiquidLevel) -> Memory/1, LL2/1
  Control/2(LiquidOut) -> TankModel/2(LiquidOut)
  Memory/1 -> Control/6(LiquidLevel)
  MR2/1 -> Control/2(ManualReference)
  CT2/1 -> Control/1(ControlType)
  F2/1 -> Control/3(Fill)
  E2/1 -> Control/4(Empty)
  EB2/1 -> Control/5(EmergencyButton)
  Control/1(LiquidIn) -> TankModel/1(LiquidIn)

== system c00017M_harness/M129/Tank2 ==
  CT2 : Inport
  F2 : Inport  Port=2
  E2 : Inport  Port=3
  MR2 : Inport  Port=4
  T2 : Inport  Port=5
  EB2 : Inport  Port=6
  Control : Subsystem
  Memory : Memory
  TankModel : Subsystem
  LL2 : Outport
  wires:
  TankModel/1(LiquidLevel) -> Memory/1, LL2/1
  Control/2(LiquidOut) -> TankModel/2(LiquidOut)
  Memory/1 -> Control/6(LiquidLevel)
  MR2/1 -> Control/2(ManualReference)
  CT2/1 -> Control/1(ControlType)
  F2/1 -> Control/3(Fill)
  E2/1 -> Control/4(Empty)
  EB2/1 -> Control/5(EmergencyButton)
  Control/1(LiquidIn) -> TankModel/1(LiquidIn)

== system c00017M_harness/M130/Tank2 ==
  CT2 : Inport
  F2 : Inport  Port=2
  E2 : Inport  Port=3
  MR2 : Inport  Port=4
  T2 : Inport  Port=5
  EB2 : Inport  Port=6
  Control : Subsystem
  Memory : Memory
  TankModel : Subsystem
  LL2 : Outport
  wires:
  TankModel/1(LiquidLevel) -> Memory/1, LL2/1
  Control/2(LiquidOut) -> TankModel/2(LiquidOut)
  Memory/1 -> Control/6(LiquidLevel)
  MR2/1 -> Control/2(ManualReference)
  CT2/1 -> Control/1(ControlType)
  F2/1 -> Control/3(Fill)
  E2/1 -> Control/4(Empty)
  EB2/1 -> Control/5(EmergencyButton)
  Control/1(LiquidIn) -> TankModel/1(LiquidIn)

== system c00017M_harness/M131/Tank2 ==
  CT2 : Inport
  F2 : Inport  Port=2
  E2 : Inport  Port=3
  MR2 : Inport  Port=4
  T2 : Inport  Port=5
  EB2 : Inport  Port=6
  Control : Subsystem
  Memory : Memory
  TankModel : Subsystem
  LL2 : Outport
  wires:
  TankModel/1(LiquidLevel) -> Memory/1, LL2/1
  Control/2(LiquidOut) -> TankModel/2(LiquidOut)
  Memory/1 -> Control/6(LiquidLevel)
  MR2/1 -> Control/2(ManualReference)
  CT2/1 -> Control/1(ControlType)
  F2/1 -> Control/3(Fill)
  E2/1 -> Control/4(Empty)
  EB2/1 -> Control/5(EmergencyButton)
  Control/1(LiquidIn) -> TankModel/1(LiquidIn)

== system c00017M_harness/M132/Tank2 ==
  CT2 : Inport
  F2 : Inport  Port=2
  E2 : Inport  Port=3
  MR2 : Inport  Port=4
  T2 : Inport  Port=5
  EB2 : Inport  Port=6
  Control : Subsystem
  Memory : Memory
  TankModel : Subsystem
  LL2 : Outport
  wires:
  TankModel/1(LiquidLevel) -> Memory/1, LL2/1
  Control/2(LiquidOut) -> TankModel/2(LiquidOut)
  Memory/1 -> Control/6(LiquidLevel)
  MR2/1 -> Control/2(ManualReference)
  CT2/1 -> Control/1(ControlType)
  F2/1 -> Control/3(Fill)
  E2/1 -> Control/4(Empty)
  EB2/1 -> Control/5(EmergencyButton)
  Control/1(LiquidIn) -> TankModel/1(LiquidIn)

== system c00017M_harness/M133/Tank2 ==
  CT2 : Inport
  F2 : Inport  Port=2
  E2 : Inport  Port=3
  MR2 : Inport  Port=4
  T2 : Inport  Port=5
  EB2 : Inport  Port=6
  Control : Subsystem
  Memory : Memory
  TankModel : Subsystem
  LL2 : Outport
  wires:
  TankModel/1(LiquidLevel) -> Memory/1, LL2/1
  Control/2(LiquidOut) -> TankModel/2(LiquidOut)
  Memory/1 -> Control/6(LiquidLevel)
  MR2/1 -> Control/2(ManualReference)
  CT2/1 -> Control/1(ControlType)
  F2/1 -> Control/3(Fill)
  E2/1 -> Control/4(Empty)
  EB2/1 -> Control/5(EmergencyButton)
  Control/1(LiquidIn) -> TankModel/1(LiquidIn)

== system c00017M_harness/M134/Tank2 ==
  CT2 : Inport
  F2 : Inport  Port=2
  E2 : Inport  Port=3
  MR2 : Inport  Port=4
  T2 : Inport  Port=5
  EB2 : Inport  Port=6
  Control : Subsystem
  Memory : Memory
  TankModel : Subsystem
  LL2 : Outport
  wires:
  TankModel/1(LiquidLevel) -> Memory/1, LL2/1
  Control/2(LiquidOut) -> TankModel/2(LiquidOut)
  Memory/1 -> Control/6(LiquidLevel)
  MR2/1 -> Control/2(ManualReference)
  CT2/1 -> Control/1(ControlType)
  F2/1 -> Control/3(Fill)
  E2/1 -> Control/4(Empty)
  EB2/1 -> Control/5(EmergencyButton)
  Control/1(LiquidIn) -> TankModel/1(LiquidIn)

== system c00017M_harness/M135/Tank2 ==
  CT2 : Inport
  F2 : Inport  Port=2
  E2 : Inport  Port=3
  MR2 : Inport  Port=4
  T2 : Inport  Port=5
  EB2 : Inport  Port=6
  Control : Subsystem
  Memory : Memory
  TankModel : Subsystem
  LL2 : Outport
  wires:
  TankModel/1(LiquidLevel) -> Memory/1, LL2/1
  Control/2(LiquidOut) -> TankModel/2(LiquidOut)
  Memory/1 -> Control/6(LiquidLevel)
  MR2/1 -> Control/2(ManualReference)
  CT2/1 -> Control/1(ControlType)
  F2/1 -> Control/3(Fill)
  E2/1 -> Control/4(Empty)
  EB2/1 -> Control/5(EmergencyButton)
  Control/1(LiquidIn) -> TankModel/1(LiquidIn)

== system c00017M_harness/M136/Tank2 ==
  CT2 : Inport
  F2 : Inport  Port=2
  E2 : Inport  Port=3
  MR2 : Inport  Port=4
  T2 : Inport  Port=5
  EB2 : Inport  Port=6
  Control : Subsystem
  Memory : Memory
  TankModel : Subsystem
  LL2 : Outport
  wires:
  TankModel/1(LiquidLevel) -> Memory/1, LL2/1
  Control/2(LiquidOut) -> TankModel/2(LiquidOut)
  Memory/1 -> Control/6(LiquidLevel)
  MR2/1 -> Control/2(ManualReference)
  CT2/1 -> Control/1(ControlType)
  F2/1 -> Control/3(Fill)
  E2/1 -> Control/4(Empty)
  EB2/1 -> Control/5(EmergencyButton)
  Control/1(LiquidIn) -> TankModel/1(LiquidIn)

== system c00017M_harness/M137/Tank2 ==
  CT2 : Inport
  F2 : Inport  Port=2
  E2 : Inport  Port=3
  MR2 : Inport  Port=4
  T2 : Inport  Port=5
  EB2 : Inport  Port=6
  Control : Subsystem
  Memory : Memory
  TankModel : Subsystem
  LL2 : Outport
  wires:
  TankModel/1(LiquidLevel) -> Memory/1, LL2/1
  Control/2(LiquidOut) -> TankModel/2(LiquidOut)
  Memory/1 -> Control/6(LiquidLevel)
  MR2/1 -> Control/2(ManualReference)
  CT2/1 -> Control/1(ControlType)
  F2/1 -> Control/3(Fill)
  E2/1 -> Control/4(Empty)
  EB2/1 -> Control/5(EmergencyButton)
  Control/1(LiquidIn) -> TankModel/1(LiquidIn)

== system c00017M_harness/M138/Tank2 ==
  CT2 : Inport
  F2 : Inport  Port=2
  E2 : Inport  Port=3
  MR2 : Inport  Port=4
  T2 : Inport  Port=5
  EB2 : Inport  Port=6
  Control : Subsystem
  Memory : Memory
  TankModel : Subsystem
  LL2 : Outport
  wires:
  TankModel/1(LiquidLevel) -> Memory/1, LL2/1
  Control/2(LiquidOut) -> TankModel/2(LiquidOut)
  Memory/1 -> Control/6(LiquidLevel)
  MR2/1 -> Control/2(ManualReference)
  CT2/1 -> Control/1(ControlType)
  F2/1 -> Control/3(Fill)
  E2/1 -> Control/4(Empty)
  EB2/1 -> Control/5(EmergencyButton)
  Control/1(LiquidIn) -> TankModel/1(LiquidIn)

== system c00017M_harness/M140/Tank2 ==
  CT2 : Inport
  F2 : Inport  Port=2
  E2 : Inport  Port=3
  MR2 : Inport  Port=4
  T2 : Inport  Port=5
  EB2 : Inport  Port=6
  Control : Subsystem
  Memory : Memory
  TankModel : Subsystem
  LL2 : Outport
  wires:
  TankModel/1(LiquidLevel) -> Memory/1, LL2/1
  Control/2(LiquidOut) -> TankModel/2(LiquidOut)
  Memory/1 -> Control/6(LiquidLevel)
  MR2/1 -> Control/2(ManualReference)
  CT2/1 -> Control/1(ControlType)
  F2/1 -> Control/3(Fill)
  E2/1 -> Control/4(Empty)
  EB2/1 -> Control/5(EmergencyButton)
  Control/1(LiquidIn) -> TankModel/1(LiquidIn)

== system c00017M_harness/M141/Tank2 ==
  CT2 : Inport
  F2 : Inport  Port=2
  E2 : Inport  Port=3
  MR2 : Inport  Port=4
  T2 : Inport  Port=5
  EB2 : Inport  Port=6
  Control : Subsystem
  Memory : Memory
  TankModel : Subsystem
  LL2 : Outport
  wires:
  TankModel/1(LiquidLevel) -> Memory/1, LL2/1
  Control/2(LiquidOut) -> TankModel/2(LiquidOut)
  Memory/1 -> Control/6(LiquidLevel)
  MR2/1 -> Control/2(ManualReference)
  CT2/1 -> Control/1(ControlType)
  F2/1 -> Control/3(Fill)
  E2/1 -> Control/4(Empty)
  EB2/1 -> Control/5(EmergencyButton)
  Control/1(LiquidIn) -> TankModel/1(LiquidIn)

== system c00017M_harness/M142/Tank2 ==
  CT2 : Inport
  F2 : Inport  Port=2
  E2 : Inport  Port=3
  MR2 : Inport  Port=4
  T2 : Inport  Port=5
  EB2 : Inport  Port=6
  Control : Subsystem
  Memory : Memory
  TankModel : Subsystem
  LL2 : Outport
  wires:
  TankModel/1(LiquidLevel) -> Memory/1, LL2/1
  Control/2(LiquidOut) -> TankModel/2(LiquidOut)
  Memory/1 -> Control/6(LiquidLevel)
  MR2/1 -> Control/2(ManualReference)
  CT2/1 -> Control/1(ControlType)
  F2/1 -> Control/3(Fill)
  E2/1 -> Control/4(Empty)
  EB2/1 -> Control/5(EmergencyButton)
  Control/1(LiquidIn) -> TankModel/1(LiquidIn)

== system c00017M_harness/M143/Tank2 ==
  CT2 : Inport
  F2 : Inport  Port=2
  E2 : Inport  Port=3
  MR2 : Inport  Port=4
  T2 : Inport  Port=5
  EB2 : Inport  Port=6
  Control : Subsystem
  Memory : Memory
  TankModel : Subsystem
  LL2 : Outport
  wires:
  TankModel/1(LiquidLevel) -> Memory/1, LL2/1
  Control/2(LiquidOut) -> TankModel/2(LiquidOut)
  Memory/1 -> Control/6(LiquidLevel)
  MR2/1 -> Control/2(ManualReference)
  CT2/1 -> Control/1(ControlType)
  F2/1 -> Control/3(Fill)
  E2/1 -> Control/4(Empty)
  EB2/1 -> Control/5(EmergencyButton)
  Control/1(LiquidIn) -> TankModel/1(LiquidIn)

== system c00017M_harness/M151/Tank2 ==
  CT2 : Inport
  F2 : Inport  Port=2
  E2 : Inport  Port=3
  MR2 : Inport  Port=4
  T2 : Inport  Port=5
  EB2 : Inport  Port=6
  Control : Subsystem
  Memory : Memory
  TankModel : Subsystem
  LL2 : Outport
  wires:
  TankModel/1(LiquidLevel) -> Memory/1, LL2/1
  Control/2(LiquidOut) -> TankModel/2(LiquidOut)
  Memory/1 -> Control/6(LiquidLevel)
  MR2/1 -> Control/2(ManualReference)
  CT2/1 -> Control/1(ControlType)
  F2/1 -> Control/3(Fill)
  E2/1 -> Control/4(Empty)
  EB2/1 -> Control/5(EmergencyButton)
  Control/1(LiquidIn) -> TankModel/1(LiquidIn)

== system c00017M_harness/M152/Tank2 ==
  CT2 : Inport
  F2 : Inport  Port=2
  E2 : Inport  Port=3
  MR2 : Inport  Port=4
  T2 : Inport  Port=5
  EB2 : Inport  Port=6
  Control : Subsystem
  Memory : Memory
  TankModel : Subsystem
  LL2 : Outport
  wires:
  TankModel/1(LiquidLevel) -> Memory/1, LL2/1
  Control/2(LiquidOut) -> TankModel/2(LiquidOut)
  Memory/1 -> Control/6(LiquidLevel)
  MR2/1 -> Control/2(ManualReference)
  CT2/1 -> Control/1(ControlType)
  F2/1 -> Control/3(Fill)
  E2/1 -> Control/4(Empty)
  EB2/1 -> Control/5(EmergencyButton)
  Control/1(LiquidIn) -> TankModel/1(LiquidIn)

== system c00017M_harness/M153/Tank2 ==
  CT2 : Inport
  F2 : Inport  Port=2
  E2 : Inport  Port=3
  MR2 : Inport  Port=4
  T2 : Inport  Port=5
  EB2 : Inport  Port=6
  Control : Subsystem
  Memory : Memory
  TankModel : Subsystem
  LL2 : Outport
  wires:
  TankModel/1(LiquidLevel) -> Memory/1, LL2/1
  Control/2(LiquidOut) -> TankModel/2(LiquidOut)
  Memory/1 -> Control/6(LiquidLevel)
  MR2/1 -> Control/2(ManualReference)
  CT2/1 -> Control/1(ControlType)
  F2/1 -> Control/3(Fill)
  E2/1 -> Control/4(Empty)
  EB2/1 -> Control/5(EmergencyButton)
  Control/1(LiquidIn) -> TankModel/1(LiquidIn)

== system c00017M_harness/M154/Tank2 ==
  CT2 : Inport
  F2 : Inport  Port=2
  E2 : Inport  Port=3
  MR2 : Inport  Port=4
  T2 : Inport  Port=5
  EB2 : Inport  Port=6
  Control : Subsystem
  Memory : Memory
  TankModel : Subsystem
  LL2 : Outport
  wires:
  TankModel/1(LiquidLevel) -> Memory/1, LL2/1
  Control/2(LiquidOut) -> TankModel/2(LiquidOut)
  Memory/1 -> Control/6(LiquidLevel)
  MR2/1 -> Control/2(ManualReference)
  CT2/1 -> Control/1(ControlType)
  F2/1 -> Control/3(Fill)
  E2/1 -> Control/4(Empty)
  EB2/1 -> Control/5(EmergencyButton)
  Control/1(LiquidIn) -> TankModel/1(LiquidIn)

== system c00017M_harness/M155/Tank2 ==
  CT2 : Inport
  F2 : Inport  Port=2
  E2 : Inport  Port=3
  MR2 : Inport  Port=4
  T2 : Inport  Port=5
  EB2 : Inport  Port=6
  Control : Subsystem
  Memory : Memory
  TankModel : Subsystem
  LL2 : Outport
  wires:
  TankModel/1(LiquidLevel) -> Memory/1, LL2/1
  Control/2(LiquidOut) -> TankModel/2(LiquidOut)
  Memory/1 -> Control/6(LiquidLevel)
  MR2/1 -> Control/2(ManualReference)
  CT2/1 -> Control/1(ControlType)
  F2/1 -> Control/3(Fill)
  E2/1 -> Control/4(Empty)
  EB2/1 -> Control/5(EmergencyButton)
  Control/1(LiquidIn) -> TankModel/1(LiquidIn)

== system c00017M_harness/M156/Tank2 ==
  CT2 : Inport
  F2 : Inport  Port=2
  E2 : Inport  Port=3
  MR2 : Inport  Port=4
  T2 : Inport  Port=5
  EB2 : Inport  Port=6
  Control : Subsystem
  Memory : Memory
  TankModel : Subsystem
  LL2 : Outport
  wires:
  TankModel/1(LiquidLevel) -> Memory/1, LL2/1
  Control/2(LiquidOut) -> TankModel/2(LiquidOut)
  Memory/1 -> Control/6(LiquidLevel)
  MR2/1 -> Control/2(ManualReference)
  CT2/1 -> Control/1(ControlType)
  F2/1 -> Control/3(Fill)
  E2/1 -> Control/4(Empty)
  EB2/1 -> Control/5(EmergencyButton)
  Control/1(LiquidIn) -> TankModel/1(LiquidIn)

== system c00017M_harness/M157/Tank2 ==
  CT2 : Inport
  F2 : Inport  Port=2
  E2 : Inport  Port=3
  MR2 : Inport  Port=4
  T2 : Inport  Port=5
  EB2 : Inport  Port=6
  Control : Subsystem
  Memory : Memory
  TankModel : Subsystem
  LL2 : Outport
  wires:
  TankModel/1(LiquidLevel) -> Memory/1, LL2/1
  Control/2(LiquidOut) -> TankModel/2(LiquidOut)
  Memory/1 -> Control/6(LiquidLevel)
  MR2/1 -> Control/2(ManualReference)
  CT2/1 -> Control/1(ControlType)
  F2/1 -> Control/3(Fill)
  E2/1 -> Control/4(Empty)
  EB2/1 -> Control/5(EmergencyButton)
  Control/1(LiquidIn) -> TankModel/1(LiquidIn)

== system c00017M_harness/M158/Tank2 ==
  CT2 : Inport
  F2 : Inport  Port=2
  E2 : Inport  Port=3
  MR2 : Inport  Port=4
  T2 : Inport  Port=5
  EB2 : Inport  Port=6
  Control : Subsystem
  Memory : Memory
  TankModel : Subsystem
  LL2 : Outport
  wires:
  TankModel/1(LiquidLevel) -> Memory/1, LL2/1
  Control/2(LiquidOut) -> TankModel/2(LiquidOut)
  Memory/1 -> Control/6(LiquidLevel)
  MR2/1 -> Control/2(ManualReference)
  CT2/1 -> Control/1(ControlType)
  F2/1 -> Control/3(Fill)
  E2/1 -> Control/4(Empty)
  EB2/1 -> Control/5(EmergencyButton)
  Control/1(LiquidIn) -> TankModel/1(LiquidIn)

== system c00017M_harness/M159/Tank2 ==
  CT2 : Inport
  F2 : Inport  Port=2
  E2 : Inport  Port=3
  MR2 : Inport  Port=4
  T2 : Inport  Port=5
  EB2 : Inport  Port=6
  Control : Subsystem
  Memory : Memory
  TankModel : Subsystem
  LL2 : Outport
  wires:
  TankModel/1(LiquidLevel) -> Memory/1, LL2/1
  Control/2(LiquidOut) -> TankModel/2(LiquidOut)
  Memory/1 -> Control/6(LiquidLevel)
  MR2/1 -> Control/2(ManualReference)
  CT2/1 -> Control/1(ControlType)
  F2/1 -> Control/3(Fill)
  E2/1 -> Control/4(Empty)
  EB2/1 -> Control/5(EmergencyButton)
  Control/1(LiquidIn) -> TankModel/1(LiquidIn)

== system c00017M_harness/M160/Tank2 ==
  CT2 : Inport
  F2 : Inport  Port=2
  E2 : Inport  Port=3
  MR2 : Inport  Port=4
  T2 : Inport  Port=5
  EB2 : Inport  Port=6
  Control : Subsystem
  Memory : Memory
  TankModel : Subsystem
  LL2 : Outport
  wires:
  TankModel/1(LiquidLevel) -> Memory/1, LL2/1
  Control/2(LiquidOut) -> TankModel/2(LiquidOut)
  Memory/1 -> Control/6(LiquidLevel)
  MR2/1 -> Control/2(ManualReference)
  CT2/1 -> Control/1(ControlType)
  F2/1 -> Control/3(Fill)
  E2/1 -> Control/4(Empty)
  EB2/1 -> Control/5(EmergencyButton)
  Control/1(LiquidIn) -> TankModel/1(LiquidIn)

== system c00017M_harness/M161/Tank2 ==
  CT2 : Inport
  F2 : Inport  Port=2
  E2 : Inport  Port=3
  MR2 : Inport  Port=4
  T2 : Inport  Port=5
  EB2 : Inport  Port=6
  Control : Subsystem
  Memory : Memory
  TankModel : Subsystem
  LL2 : Outport
  wires:
  TankModel/1(LiquidLevel) -> Memory/1, LL2/1
  Control/2(LiquidOut) -> TankModel/2(LiquidOut)
  Memory/1 -> Control/6(LiquidLevel)
  MR2/1 -> Control/2(ManualReference)
  CT2/1 -> Control/1(ControlType)
  F2/1 -> Control/3(Fill)
  E2/1 -> Control/4(Empty)
  EB2/1 -> Control/5(EmergencyButton)
  Control/1(LiquidIn) -> TankModel/1(LiquidIn)
